simulink library "BibFHDO"  (R2025b)
settings: Solver=VariableStepAuto  StartTime=0.0  StopTime=10.0  RelTol=1e-3
libraries: $bdroot x16, BibSpielo x3, Bibliothek_FHDO_V1 x2
settings Model: Creator=henni  LastModifiedBy=henni

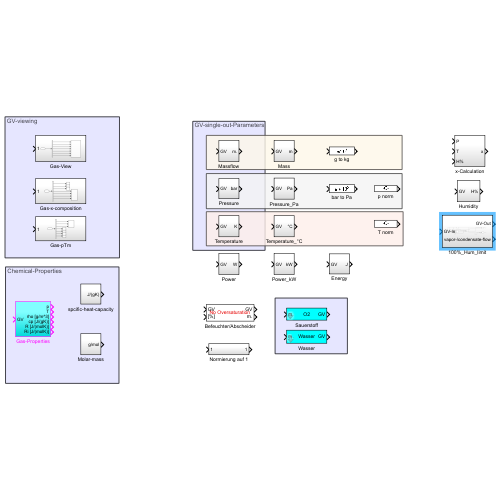
[thumbnail: Simulink's stored preview of the top-level diagram]
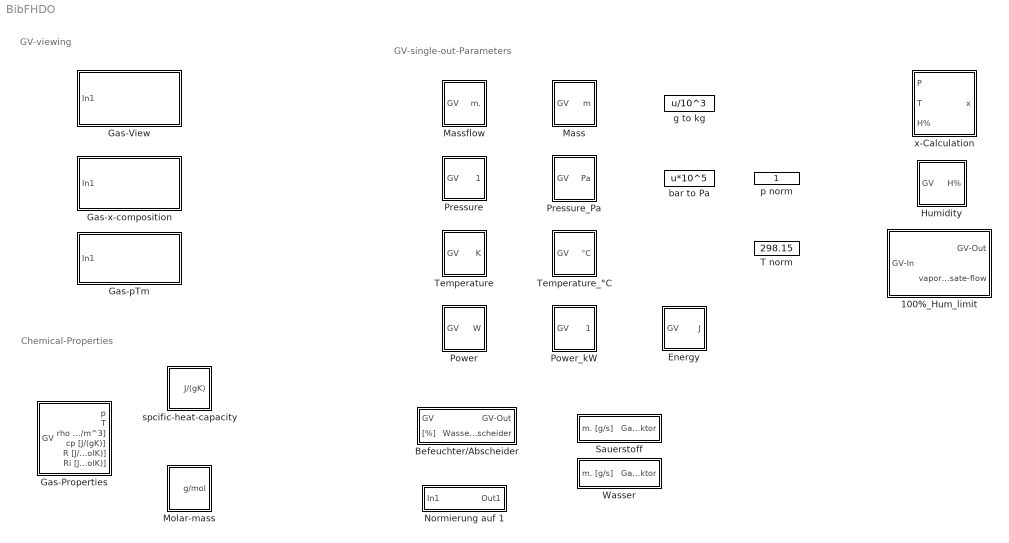
== system BibFHDO ==
  note: Chemical-Properties
  note: GV-viewing
  note: GV-single-out-Parameters
  100%_Hum_limit : Subsystem
  Befeuchter/Abscheider : Subsystem
      mask Display:
      | color('red')
      | disp('No Oversaturation');
      | 
      | color('black')
      | port_label('output', 1, 'GV')
      | port_label('output', 2, 'm.')
      | port_label('input', 1, 'GV')
      | port_label('input', 2, '[%]')
  Energy : Subsystem
  Gas-Properties : Subsystem
  Gas-View : Subsystem
  Gas-pTm : Subsystem
  Gas-x-composition : Subsystem
  Humidity : Subsystem
  Mass : Subsystem
  Massflow : Subsystem
  Molar-mass : Subsystem
  Normierung auf 1 : Subsystem
  Power : Subsystem
  Power_kW : Subsystem
  Pressure : Subsystem
  Pressure_Pa : Subsystem
  Sauerstoff : Subsystem  mask{p=1, T=25}
      mask prompts: p "p [bar]"; T "T [°C]"
      mask Display:
      | disp('O2')
      | 
      | port_label ('input', 1, 'm.')
      | port_label ('output', 1, 'GV')
  T norm : Constant  Value=298.15
  Temperature : Subsystem
  Temperature_°C : Subsystem
  Wasser : Subsystem  mask{p=1, T=25}
      mask prompts: p "p [bar]"; T "T [°C]"
      mask Display:
      | disp('Wasser')
      | 
      | port_label ('input', 1, 'm.')
      | port_label ('output', 1, 'GV')
  bar to Pa : Fcn  Expr=u*10^5
  g to kg : Fcn  Expr=u/10^3
  p norm : Constant
  spcific-heat-capacity : Subsystem
  x-Calculation : Subsystem

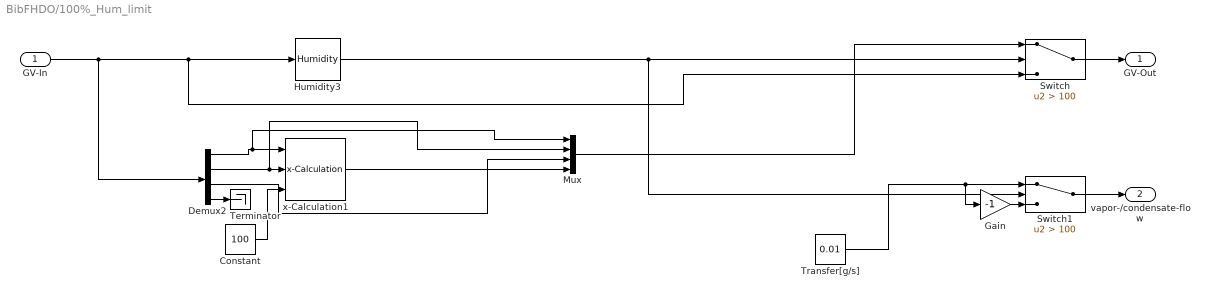
== system BibFHDO/100%_Hum_limit ==
  GV-In : Inport
  Constant : Constant  Value=100
  Demux2 : Demux  Outputs=[1 1 1 4]
  Gain : Gain  Gain=-1
  Humidity3 : $bdroot/Humidity  SystemSampleTime=-1  VariantActivationTime=update diagram  EmptyChoice=off  PassThrough=off  PassThroughVariantControl=(default)  EmptyChoiceVariantControl=(default)  AllowFlexibleInterface=on  Latency=0  AutoFrameSizeCalculation=off
  Mux : Mux  Inputs=[1 1 1 4]
  Switch : Switch  Criteria=u2 > Threshold  Threshold=100  SaturateOnIntegerOverflow=off  InputSameDT=off
  Switch1 : Switch  Criteria=u2 > Threshold  Threshold=100  SaturateOnIntegerOverflow=off  InputSameDT=off
  Terminator : Terminator
  Transfer[g/s] : Constant  Value=0.01
  x-Calculation1 : $bdroot/x-Calculation  SystemSampleTime=-1  VariantActivationTime=update diagram  EmptyChoice=off  PassThrough=off  PassThroughVariantControl=(default)  EmptyChoiceVariantControl=(default)  AllowFlexibleInterface=on  Latency=0  AutoFrameSizeCalculation=off
  GV-Out : Outport
  vapor-/condensate-flow : Outport  Port=2
  wires:
  Transfer[g/s]/1 -> Gain/1, Switch1/1
  Gain/1 -> Switch1/3
  Switch1/1 -> vapor-/condensate-flow/1
  x-Calculation1/1 -> Mux/4
  Switch/1 -> GV-Out/1
  Demux2/1 -> x-Calculation1/1, Mux/1
  Demux2/3 -> Mux/3
  Demux2/4 -> Terminator/1
  Demux2/2 -> x-Calculation1/2, Mux/2
  Humidity3/1 -> Switch/2, Switch1/2
  GV-In/1 -> Switch/3, Humidity3/1, Demux2/1
  Mux/1 -> Switch/1
  Constant/1 -> x-Calculation1/3

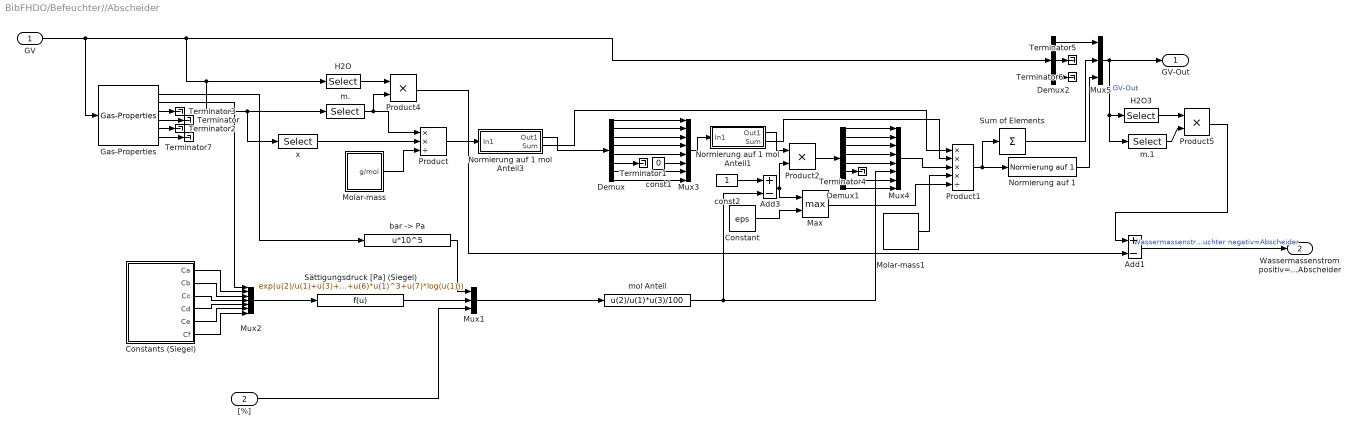
== system BibFHDO/Befeuchter//Abscheider ==
  GV : Inport
  "[%]" : Inport  Port=2
  Add1 : Sum  Inputs=+-
  Add3 : Sum  Inputs=+-
  Constant : Constant  Value=eps
  Constants (Siegel) : Subsystem
  Demux : Demux  Outputs=8
  Demux1 : Demux  Outputs=8
  Demux2 : Demux  Outputs=[2 1 8]
  Gas-Properties : $bdroot/Gas-Properties  SystemSampleTime=-1  VariantActivationTime=update diagram  EmptyChoice=off  PassThrough=off  PassThroughVariantControl=(default)  EmptyChoiceVariantControl=(default)  AllowFlexibleInterface=on  Latency=0  AutoFrameSizeCalculation=off
  H2O : Selector  InputPortWidth=11  IndexOptions=Index vector (dialog)  Indices=9  OutputSizes=1
  H2O3 : Selector  InputPortWidth=11  IndexOptions=Index vector (dialog)  Indices=9  OutputSizes=1
  Max : MinMax  Function=max  Inputs=2
  Molar-mass : Subsystem
  Molar-mass1 : $bdroot/Molar-mass  SystemSampleTime=-1  VariantActivationTime=update diagram  EmptyChoice=off  PassThrough=off  PassThroughVariantControl=(default)  EmptyChoiceVariantControl=(default)  AllowFlexibleInterface=on  Latency=0  AutoFrameSizeCalculation=off
  Mux1 : Mux  Inputs=3
  Mux2 : Mux  Inputs=7
  Mux3 : Mux  Inputs=8
  Mux4 : Mux  Inputs=8
  Mux5 : Mux  Inputs=3
  Normierung auf 1 : $bdroot/Normierung auf 1  SystemSampleTime=-1  VariantActivationTime=update diagram  EmptyChoice=off  PassThrough=off  PassThroughVariantControl=(default)  EmptyChoiceVariantControl=(default)  AllowFlexibleInterface=on  Latency=0  AutoFrameSizeCalculation=off
  Normierung auf 1 mol Anteil1 : Subsystem
  Normierung auf 1 mol Anteil3 : Subsystem
  Product : Product  Inputs=**/  RndMeth=Zero
  Product1 : Product  Inputs=****/  RndMeth=Zero
  Product2 : Product  RndMeth=Zero
  Product4 : Product  RndMeth=Zero
  Product5 : Product  RndMeth=Zero
  Sum of Elements : Sum  Inputs=+
  Sättigungsdruck [Pa] (Siegel) : Fcn  Expr=exp(u(2)/u(1)+u(3)+u(4)*u(1)+u(5)*u(1)^2+u(6)*u(1)^3+u(7)*log(u(1)))
  Terminator{,1..7} (8 alike) : Terminator
  "bar -> Pa" : Fcn  Expr=u*10^5
  const1 : Constant  Value=0
  const2 : Constant
  m. : Selector  InputPortWidth=11  IndexOptions=Index vector (dialog)  Indices=3  OutputSizes=1
  m.1 : Selector  InputPortWidth=11  IndexOptions=Index vector (dialog)  Indices=3  OutputSizes=1
  mol Anteil : Fcn  Expr=u(2)/u(1)*u(3)/100
  x : Selector  InputPortWidth=11  IndexOptions=Index vector (dialog)  Indices=[4 5 6 7 8 9 10 11]  OutputSizes=1
  GV-Out : Outport
  Wassermassenstrom positiv=Befeuchter negativ=Abscheider : Outport  Port=2
  wires:
  Product1/1 -> Normierung auf 1/1, Sum of Elements/1
  Sättigungsdruck [Pa] (Siegel)/1 -> Mux1/2
  Demux1/2 -> Mux4/2
  Gas-Properties/6 -> Terminator7/1
  Constants (Siegel)/5(Ce) -> Mux2/6
  Demux/2 -> Mux3/2
  Constants (Siegel)/1(Ca) -> Mux2/2
  Demux2/1 -> Mux5/1
  Demux/3 -> Mux3/3
  Molar-mass/1(g/mol) -> Product/3
  Mux3/1 -> Normierung auf 1 mol Anteil1/1(In1)
  GV/1 -> Gas-Properties/1, Demux2/1, m./1, x/1, H2O/1
  Product4/1 -> Add1/2
  Normierung auf 1 mol Anteil1/1(Out1) -> Product2/1
  Gas-Properties/1 -> "bar -> Pa"/1
  Constants (Siegel)/6(Cf) -> Mux2/7
  Normierung auf 1/1 -> Mux5/3
  const2/1 -> Add3/1
  Demux1/4 -> Mux4/4
  Gas-Properties/2 -> Mux2/1
  Demux1/1 -> Mux4/1
  Demux1/5 -> Mux4/5
  Constants (Siegel)/2(Cb) -> Mux2/3
  Demux/8 -> Mux3/8
  Demux/6 -> Terminator1/1
  Product2/1 -> Demux1/1
  Demux/1 -> Mux3/1
  Molar-mass1/1 -> Product1/4
  Mux2/1 -> Sättigungsdruck [Pa] (Siegel)/1
  Demux1/7 -> Mux4/7
  Add3/1 -> Max/1, Product2/2
  Mux5/1 -> m.1/1, H2O3/1, GV-Out/1  "GV-Out"
  Add1/1 -> Wassermassenstrom positiv=Befeuchter negativ=Abscheider/1  "Wassermassenstrom positiv=Befeuchter negativ=Abscheider"
  Demux1/3 -> Mux4/3
  Sum of Elements/1 -> Mux5/2
  m.1/1 -> Product5/2
  Product5/1 -> Add1/1
  Product/1 -> Normierung auf 1 mol Anteil3/1(In1)
  Demux2/2 -> Terminator5/1
  Gas-Properties/3 -> Terminator3/1
  x/1 -> Product/2
  const1/1 -> Mux3/6
  H2O/1 -> Product4/1
  mol Anteil/1 -> Mux4/6, Add3/2
  Demux/7 -> Mux3/7
  H2O3/1 -> Product5/1
  Constants (Siegel)/3(Cc) -> Mux2/4
  Mux1/1 -> mol Anteil/1
  Normierung auf 1 mol Anteil1/2(Sum) -> Product1/2
  "bar -> Pa"/1 -> Mux1/1
  Demux1/6 -> Terminator4/1
  m./1 -> Product/1, Product4/2
  Mux4/1 -> Product1/3
  Demux2/3 -> Terminator6/1
  Demux1/8 -> Mux4/8
  Demux/4 -> Mux3/4
  Demux/5 -> Mux3/5
  Normierung auf 1 mol Anteil3/1(Out1) -> Demux/1
  Normierung auf 1 mol Anteil3/2(Sum) -> Product1/1
  Constants (Siegel)/4(Cd) -> Mux2/5
  Gas-Properties/4 -> Terminator/1
  Gas-Properties/5 -> Terminator2/1
  "[%]"/1 -> Mux1/3
  Constant/1 -> Max/2
  Max/1 -> Product1/5

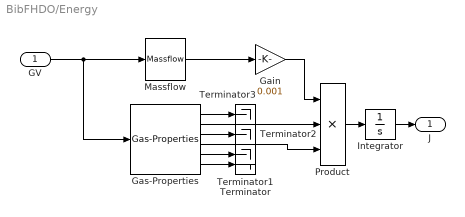
== system BibFHDO/Energy ==
  GV : Inport
  Gain : Gain  Gain=0.001
  Gas-Properties : $bdroot/Gas-Properties  SystemSampleTime=-1  VariantActivationTime=update diagram  EmptyChoice=off  PassThrough=off  PassThroughVariantControl=(default)  EmptyChoiceVariantControl=(default)  AllowFlexibleInterface=on  Latency=0  AutoFrameSizeCalculation=off
  Integrator : Integrator
  Massflow : $bdroot/Massflow  SystemSampleTime=-1  VariantActivationTime=update diagram  EmptyChoice=off  PassThrough=off  PassThroughVariantControl=(default)  EmptyChoiceVariantControl=(default)  AllowFlexibleInterface=on  Latency=0  AutoFrameSizeCalculation=off
  Product : Product  Inputs=3
  Terminator{,1..3} (4 alike) : Terminator
  J : Outport
  wires:
  GV/1 -> Gas-Properties/1, Massflow/1
  Gas-Properties/5 -> Terminator1/1
  Gas-Properties/2 -> Product/2
  Gas-Properties/3 -> Terminator2/1
  Gas-Properties/1 -> Terminator3/1
  Gas-Properties/4 -> Product/3
  Massflow/1 -> Gain/1
  Gas-Properties/6 -> Terminator/1
  Gain/1 -> Product/1
  Product/1 -> Integrator/1
  Integrator/1 -> J/1

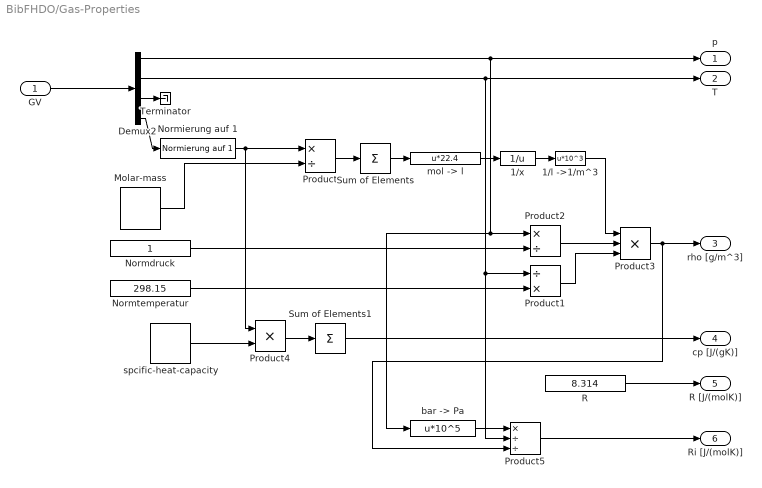
== system BibFHDO/Gas-Properties ==
  GV : Inport
  1/l ->1/m^3 : Fcn  Expr=u*10^3
  1/x : Fcn  Expr=1/u
  Demux2 : Demux  Outputs=[1 1 1 4]
  Molar-mass : BibSpielo/Molar-mass  SystemSampleTime=-1  VariantActivationTime=update diagram  EmptyChoice=off  PassThrough=off  PassThroughVariantControl=(default)  EmptyChoiceVariantControl=(default)  AllowFlexibleInterface=on  Latency=0  AutoFrameSizeCalculation=off
  Normdruck : Constant
  Normierung auf 1 : BibSpielo/Normierung auf 1  SystemSampleTime=-1  VariantActivationTime=update diagram  EmptyChoice=off  PassThrough=off  PassThroughVariantControl=(default)  EmptyChoiceVariantControl=(default)  AllowFlexibleInterface=on  Latency=0  AutoFrameSizeCalculation=off
  Normtemperatur : Constant  Value=298.15
  Product : Product  Inputs=*/  RndMeth=Zero
  Product1 : Product  Inputs=/*  RndMeth=Zero
  Product2 : Product  Inputs=*/  RndMeth=Zero
  Product3 : Product  Inputs=3  RndMeth=Zero
  Product4 : Product  RndMeth=Zero
  Product5 : Product  Inputs=*//
  R : Constant  Value=8.314
  Sum of Elements : Sum  Inputs=+
  Sum of Elements1 : Sum  Inputs=+
  Terminator : Terminator
  "bar -> Pa" : Fcn  Expr=u*10^5
  "mol -> l" : Fcn  Expr=u*22.4
  spcific-heat-capacity : BibSpielo/spcific-heat-capacity  SystemSampleTime=-1  VariantActivationTime=update diagram  EmptyChoice=off  PassThrough=off  PassThroughVariantControl=(default)  EmptyChoiceVariantControl=(default)  AllowFlexibleInterface=on  Latency=0  AutoFrameSizeCalculation=off
  p : Outport
  T : Outport  Port=2
  rho [g/m^3] : Outport  Port=3
  cp [J/(gK)] : Outport  Port=4
  R [J/(molK)] : Outport  Port=5
  Ri [J/(molK)] : Outport  Port=6
  wires:
  1/l ->1/m^3/1 -> Product3/1
  Product2/1 -> Product3/2
  1/x/1 -> 1/l ->1/m^3/1
  R/1 -> R [J/(molK)]/1
  Demux2/1 -> p/1, Product2/1, "bar -> Pa"/1
  GV/1 -> Demux2/1
  spcific-heat-capacity/1 -> Product4/2
  "mol -> l"/1 -> 1/x/1
  Product1/1 -> Product3/3
  Molar-mass/1 -> Product/2
  Normtemperatur/1 -> Product1/2
  Normierung auf 1/1 -> Product/1, Product4/1
  Sum of Elements/1 -> "mol -> l"/1
  Demux2/3 -> Terminator/1
  "bar -> Pa"/1 -> Product5/1
  Product4/1 -> Sum of Elements1/1
  Demux2/2 -> T/1, Product5/2, Product1/1
  Sum of Elements1/1 -> cp [J/(gK)]/1
  Product/1 -> Sum of Elements/1
  Product3/1 -> rho [g/m^3]/1, Product5/3
  Normdruck/1 -> Product2/2
  Demux2/4 -> Normierung auf 1/1
  Product5/1 -> Ri [J/(molK)]/1

== system BibFHDO/Gas-View ==
  In1 : Inport
  Demux : Demux  Outputs=7
  Scope : Scope  NumInputPorts=7
  wires:
  In1/1 -> Demux/1
  Demux/5 -> Scope/5  "H2O"
  Demux/6 -> Scope/6  "O2"
  Demux/4 -> Scope/4  "H2%"
  Demux/7 -> Scope/7  "N2"
  Demux/1 -> Scope/1  "Druck"
  Demux/2 -> Scope/2  "Temperatur"
  Demux/3 -> Scope/3  "Massenstrom"

== system BibFHDO/Gas-pTm ==
  In1 : Inport
  Demux : Demux  Outputs=7
  Scope : Scope  NumInputPorts=3
      settings: DataLoggingVariableName=ScopeData2
  Terminator{,1..3} (4 alike) : Terminator
  wires:
  Demux/6 -> Terminator1/1
  In1/1 -> Demux/1
  Demux/3 -> Scope/3  "m"
  Demux/1 -> Scope/1  "p"
  Demux/2 -> Scope/2  "T"
  Demux/4 -> Terminator3/1
  Demux/5 -> Terminator2/1
  Demux/7 -> Terminator/1

== system BibFHDO/Gas-x-composition ==
  In1 : Inport
  Demux : Demux  Outputs=7
  Scope : Scope  NumInputPorts=4
  Terminator : Terminator
  Terminator1 : Terminator
  Terminator2 : Terminator
  wires:
  Demux/6 -> Scope/3  "O2"
  Demux/7 -> Scope/4  "N2"
  In1/1 -> Demux/1
  Demux/2 -> Terminator1/1
  Demux/1 -> Terminator/1
  Demux/4 -> Scope/1  "H2"
  Demux/3 -> Terminator2/1
  Demux/5 -> Scope/2  "H2O"

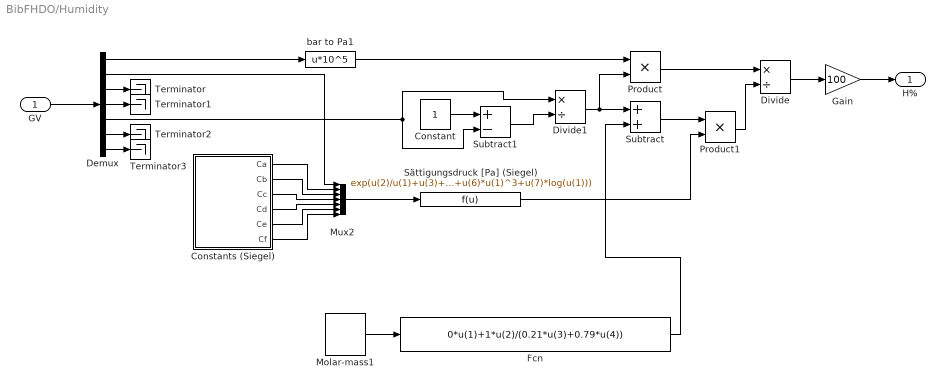
== system BibFHDO/Humidity ==
  GV : Inport
  Constant : Constant
  Constants (Siegel) : Subsystem
  Demux : Demux  Outputs=7
  Divide : Product  Inputs=*/
  Divide1 : Product  Inputs=*/
  Fcn : Fcn  Expr=0*u(1)+1*u(2)/(0.21*u(3)+0.79*u(4))
  Gain : Gain  Gain=100
  Molar-mass1 : $bdroot/Molar-mass  SystemSampleTime=-1  VariantActivationTime=update diagram  EmptyChoice=off  PassThrough=off  PassThroughVariantControl=(default)  EmptyChoiceVariantControl=(default)  AllowFlexibleInterface=on  Latency=0  AutoFrameSizeCalculation=off
  Mux2 : Mux  Inputs=7
  Product : Product
  Product1 : Product
  Subtract : Sum
  Subtract1 : Sum  Inputs=+-
  Sättigungsdruck [Pa] (Siegel) : Fcn  Expr=exp(u(2)/u(1)+u(3)+u(4)*u(1)+u(5)*u(1)^2+u(6)*u(1)^3+u(7)*log(u(1)))
  Terminator{,1..3} (4 alike) : Terminator
  bar to Pa1 : Fcn  Expr=u*10^5
  H% : Outport
  wires:
  Demux/2 -> Mux2/1
  Constants (Siegel)/2(Cb) -> Mux2/3
  Mux2/1 -> Sättigungsdruck [Pa] (Siegel)/1
  Fcn/1 -> Subtract/2
  Demux/5 -> Divide1/1, Subtract1/2
  GV/1 -> Demux/1
  Demux/6 -> Terminator2/1
  Demux/3 -> Terminator/1
  Molar-mass1/1 -> Fcn/1
  bar to Pa1/1 -> Product/1
  Divide/1 -> Gain/1
  Demux/1 -> bar to Pa1/1
  Demux/4 -> Terminator1/1
  Demux/7 -> Terminator3/1
  Constants (Siegel)/4(Cd) -> Mux2/5
  Constants (Siegel)/6(Cf) -> Mux2/7
  Constants (Siegel)/3(Cc) -> Mux2/4
  Constants (Siegel)/5(Ce) -> Mux2/6
  Constants (Siegel)/1(Ca) -> Mux2/2
  Product/1 -> Divide/1
  Subtract/1 -> Product1/1
  Sättigungsdruck [Pa] (Siegel)/1 -> Product1/2
  Product1/1 -> Divide/2
  Gain/1 -> H%/1
  Constant/1 -> Subtract1/1
  Subtract1/1 -> Divide1/2
  Divide1/1 -> Product/2, Subtract/1

== system BibFHDO/Mass ==
  GV : Inport
  Integrator : Integrator
  Massflow : $bdroot/Massflow  SystemSampleTime=-1  VariantActivationTime=update diagram  EmptyChoice=off  PassThrough=off  PassThroughVariantControl=(default)  EmptyChoiceVariantControl=(default)  AllowFlexibleInterface=on  Latency=0  AutoFrameSizeCalculation=off
  m : Outport
  wires:
  Massflow/1 -> Integrator/1
  GV/1 -> Massflow/1
  Integrator/1 -> m/1

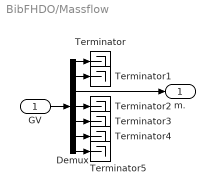
== system BibFHDO/Massflow ==
  GV : Inport
  Demux : Demux  Outputs=7
  Terminator{,1..5} (6 alike) : Terminator
  m. : Outport
  wires:
  Demux/2 -> Terminator1/1
  GV/1 -> Demux/1
  Demux/4 -> Terminator2/1
  Demux/6 -> Terminator4/1
  Demux/5 -> Terminator3/1
  Demux/1 -> Terminator/1
  Demux/7 -> Terminator5/1
  Demux/3 -> m./1

== system BibFHDO/Molar-mass ==
  note: VDI Wärmeatlas
      | Normbedingungen
      | p=1bar
      | T=298.15K
  H2 : Constant  Value=2.016
  H2O : Constant  Value=18.015
  Mux : Mux
  N2 : Constant  Value=28.013
  O2 : Constant  Value=31.999
  g/mol : Outport
  wires:
  H2O/1 -> Mux/2
  N2/1 -> Mux/4
  O2/1 -> Mux/3
  Mux/1 -> g/mol/1
  H2/1 -> Mux/1

== system BibFHDO/Normierung auf 1 ==
  In1 : Inport
  Product : Product  Inputs=*/  RndMeth=Zero
  Sum of Elements : Sum  Inputs=+
  Out1 : Outport
  wires:
  Sum of Elements/1 -> Product/2
  In1/1 -> Product/1, Sum of Elements/1
  Product/1 -> Out1/1

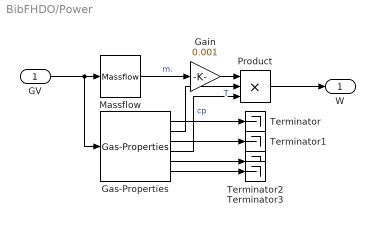
== system BibFHDO/Power ==
  GV : Inport
  Gain : Gain  Gain=0.001
  Gas-Properties : $bdroot/Gas-Properties  SystemSampleTime=-1  VariantActivationTime=update diagram  EmptyChoice=off  PassThrough=off  PassThroughVariantControl=(default)  EmptyChoiceVariantControl=(default)  AllowFlexibleInterface=on  Latency=0  AutoFrameSizeCalculation=off
  Massflow : $bdroot/Massflow  SystemSampleTime=-1  VariantActivationTime=update diagram  EmptyChoice=off  PassThrough=off  PassThroughVariantControl=(default)  EmptyChoiceVariantControl=(default)  AllowFlexibleInterface=on  Latency=0  AutoFrameSizeCalculation=off
  Product : Product  Inputs=3
  Terminator{,1..3} (4 alike) : Terminator
  W : Outport
  wires:
  Massflow/1 -> Gain/1  "m."
  Gas-Properties/3 -> Terminator1/1
  GV/1 -> Gas-Properties/1, Massflow/1
  Gas-Properties/2 -> Product/2  "T"
  Gas-Properties/1 -> Terminator/1
  Gas-Properties/4 -> Product/3  "cp"
  Gas-Properties/5 -> Terminator2/1
  Gas-Properties/6 -> Terminator3/1
  Product/1 -> W/1
  Gain/1 -> Product/1

== system BibFHDO/Power_kW ==
  GV : Inport
  Gain : Gain  Gain=1000
  Power : $bdroot/Power  SystemSampleTime=-1  VariantActivationTime=update diagram  EmptyChoice=off  PassThrough=off  PassThroughVariantControl=(default)  EmptyChoiceVariantControl=(default)  AllowFlexibleInterface=on  Latency=0  AutoFrameSizeCalculation=off
  kW : Outport
  wires:
  GV/1 -> Power/1
  Gain/1 -> kW/1
  Power/1 -> Gain/1

== system BibFHDO/Pressure ==
  GV : Inport
  Demux : Demux  Outputs=7
  Terminator{1..6} (6 alike) : Terminator
  bar : Outport
  wires:
  Demux/3 -> Terminator6/1
  Demux/7 -> Terminator5/1
  Demux/6 -> Terminator4/1
  GV/1 -> Demux/1
  Demux/4 -> Terminator2/1
  Demux/2 -> Terminator1/1
  Demux/5 -> Terminator3/1
  Demux/1 -> bar/1

== system BibFHDO/Pressure_Pa ==
  GV : Inport
  Multiply : Gain  Gain=100000
  Pressure : $bdroot/Pressure  SystemSampleTime=-1  VariantActivationTime=update diagram  EmptyChoice=off  PassThrough=off  PassThroughVariantControl=(default)  EmptyChoiceVariantControl=(default)  AllowFlexibleInterface=on  Latency=0  AutoFrameSizeCalculation=off
  Pa : Outport
  wires:
  Pressure/1 -> Multiply/1
  GV/1 -> Pressure/1
  Multiply/1 -> Pa/1

== system BibFHDO/Sauerstoff ==
  m. [g/s] : Inport
  Mux : Mux
  Normierung auf 2 : Bibliothek_FHDO_V1/Sauerstoff/Normierung auf 1  SystemSampleTime=-1  VariantActivationTime=update diagram  EmptyChoice=off  PassThrough=off  PassThroughVariantControl=(default)  EmptyChoiceVariantControl=(default)  AllowFlexibleInterface=on  Latency=0  AutoFrameSizeCalculation=off
  Saturation : Saturate  UpperLimit=inf  LowerLimit=eps
  T : Constant  Value=273.15+T
  p : Constant  Value=p
  x : Constant  Value=[0 0 1 0]
  Gasvektor : Outport
  wires:
  p/1 -> Mux/1
  x/1 -> Normierung auf 2/1
  Normierung auf 2/1 -> Mux/4
  Mux/1 -> Gasvektor/1  "Gasvektor"
  T/1 -> Mux/2
  m. [g/s]/1 -> Saturation/1
  Saturation/1 -> Mux/3

== system BibFHDO/Temperature ==
  GV : Inport
  Demux : Demux  Outputs=7
  Terminator{,1..5} (6 alike) : Terminator
  K : Outport
  wires:
  Demux/3 -> Terminator1/1
  Demux/7 -> Terminator5/1
  GV/1 -> Demux/1
  Demux/4 -> Terminator2/1
  Demux/1 -> Terminator/1
  Demux/6 -> Terminator4/1
  Demux/5 -> Terminator3/1
  Demux/2 -> K/1

== system BibFHDO/Temperature_°C ==
  GV : Inport
  Add Constant : Bias  Bias=273.15  SaturateOnIntegerOverflow=off
  Temperature : $bdroot/Temperature  SystemSampleTime=-1  VariantActivationTime=update diagram  EmptyChoice=off  PassThrough=off  PassThroughVariantControl=(default)  EmptyChoiceVariantControl=(default)  AllowFlexibleInterface=on  Latency=0  AutoFrameSizeCalculation=off
  °C : Outport
  wires:
  GV/1 -> Temperature/1
  Temperature/1 -> Add Constant/1
  Add Constant/1 -> °C/1

== system BibFHDO/Wasser ==
  m. [g/s] : Inport
  Mux : Mux
  Normierung auf 2 : Bibliothek_FHDO_V1/Wasser/Normierung auf 1  SystemSampleTime=-1  VariantActivationTime=update diagram  EmptyChoice=off  PassThrough=off  PassThroughVariantControl=(default)  EmptyChoiceVariantControl=(default)  AllowFlexibleInterface=on  Latency=0  AutoFrameSizeCalculation=off
  Saturation : Saturate  UpperLimit=inf  LowerLimit=eps
  T : Constant  Value=273.15+T
  p : Constant  Value=p
  x : Constant  Value=[0 1 0 0]
  Gasvektor : Outport
  wires:
  p/1 -> Mux/1
  T/1 -> Mux/2
  Normierung auf 2/1 -> Mux/4
  Saturation/1 -> Mux/3
  x/1 -> Normierung auf 2/1
  Mux/1 -> Gasvektor/1  "Gasvektor"
  m. [g/s]/1 -> Saturation/1

== system BibFHDO/spcific-heat-capacity ==
  note: VDI Wärmeatlas
      | Normbedingungen
      | p=1bar
      | T=298.15K
  H2 : Constant  Value=14.286
  H2O : Constant  Value=1.879
  Mux : Mux
  N2 : Constant  Value=1.037
  O2 : Constant  Value=0.927
  J/(gK) : Outport
  wires:
  N2/1 -> Mux/4
  H2O/1 -> Mux/2
  O2/1 -> Mux/3
  Mux/1 -> J/(gK)/1
  H2/1 -> Mux/1

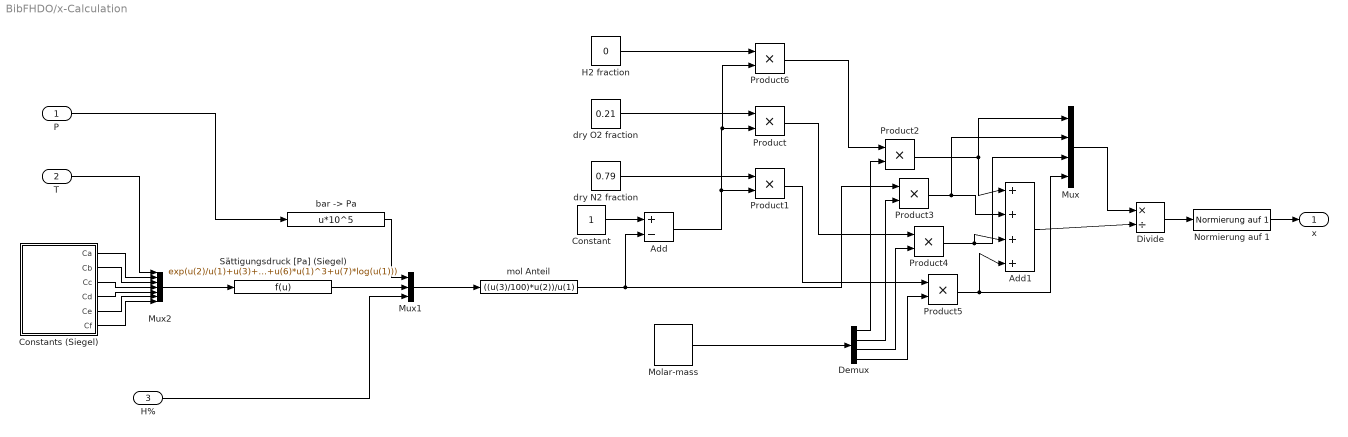
== system BibFHDO/x-Calculation ==
  P : Inport
  T : Inport  Port=2
  H% : Inport  Port=3
  Add : Sum  Inputs=+-
  Add1 : Sum  Inputs=++++
  Constant : Constant
  Constants (Siegel) : Subsystem
  Demux : Demux
  Divide : Product  Inputs=*/
  H2 fraction : Constant  Value=0
  Molar-mass : $bdroot/Molar-mass  SystemSampleTime=-1  VariantActivationTime=update diagram  EmptyChoice=off  PassThrough=off  PassThroughVariantControl=(default)  EmptyChoiceVariantControl=(default)  AllowFlexibleInterface=on  Latency=0  AutoFrameSizeCalculation=off
  Mux : Mux
  Mux1 : Mux  Inputs=3
  Mux2 : Mux  Inputs=7
  Normierung auf 1 : $bdroot/Normierung auf 1  SystemSampleTime=-1  VariantActivationTime=update diagram  EmptyChoice=off  PassThrough=off  PassThroughVariantControl=(default)  EmptyChoiceVariantControl=(default)  AllowFlexibleInterface=on  Latency=0  AutoFrameSizeCalculation=off
  Product{,1..6} (7 alike) : Product
  Sättigungsdruck [Pa] (Siegel) : Fcn  Expr=exp(u(2)/u(1)+u(3)+u(4)*u(1)+u(5)*u(1)^2+u(6)*u(1)^3+u(7)*log(u(1)))
  "bar -> Pa" : Fcn  Expr=u*10^5
  dry N2 fraction : Constant  Value=0.79
  dry O2 fraction : Constant  Value=0.21
  mol Anteil : Fcn  Expr=((u(3)/100)*u(2))/u(1)
  x : Outport
  wires:
  Constants (Siegel)/4(Cd) -> Mux2/5
  Constants (Siegel)/3(Cc) -> Mux2/4
  Constants (Siegel)/6(Cf) -> Mux2/7
  Constants (Siegel)/5(Ce) -> Mux2/6
  Constants (Siegel)/1(Ca) -> Mux2/2
  "bar -> Pa"/1 -> Mux1/1
  Sättigungsdruck [Pa] (Siegel)/1 -> Mux1/2
  Mux2/1 -> Sättigungsdruck [Pa] (Siegel)/1
  Constants (Siegel)/2(Cb) -> Mux2/3
  Mux1/1 -> mol Anteil/1
  H%/1 -> Mux1/3
  mol Anteil/1 -> Product3/1, Add/2
  P/1 -> "bar -> Pa"/1
  dry O2 fraction/1 -> Product/1
  dry N2 fraction/1 -> Product1/1
  Constant/1 -> Add/1
  H2 fraction/1 -> Product6/1
  Product1/1 -> Product5/1
  Product/1 -> Product4/1
  Molar-mass/1 -> Demux/1
  Demux/1 -> Product2/2
  Demux/2 -> Product3/2
  Demux/4 -> Product5/2
  Demux/3 -> Product4/2
  Product2/1 -> Mux/1, Add1/1
  Product3/1 -> Mux/2, Add1/2
  Product4/1 -> Mux/3, Add1/3
  Product5/1 -> Mux/4, Add1/4
  Mux/1 -> Divide/1
  Divide/1 -> Normierung auf 1/1
  Add1/1 -> Divide/2
  T/1 -> Mux2/1
  Normierung auf 1/1 -> x/1
  Product6/1 -> Product2/1
  Add/1 -> Product6/2, Product/2, Product1/2

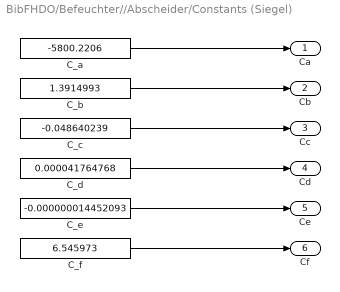
== system BibFHDO/Befeuchter//Abscheider/Constants (Siegel) ==
  C_a : Constant  Value=-5800.2206
  C_b : Constant  Value=1.3914993
  C_c : Constant  Value=-0.048640239
  C_d : Constant  Value=0.000041764768
  C_e : Constant  Value=-0.000000014452093
  C_f : Constant  Value=6.545973
  Ca : Outport
  Cb : Outport  Port=2
  Cc : Outport  Port=3
  Cd : Outport  Port=4
  Ce : Outport  Port=5
  Cf : Outport  Port=6
  wires:
  C_f/1 -> Cf/1
  C_a/1 -> Ca/1
  C_e/1 -> Ce/1
  C_d/1 -> Cd/1
  C_c/1 -> Cc/1
  C_b/1 -> Cb/1

== system BibFHDO/Befeuchter//Abscheider/Molar-mass ==
  note: VDI Wärmeatlas
      | Normbedingungen
      | p=1bar
      | T=298.15K
  H2 : Constant  Value=2.016
  H2O : Constant  Value=18.015
  Mux : Mux
  N2 : Constant  Value=28.013
  O2 : Constant  Value=31.999
  g/mol : Outport
  wires:
  H2O/1 -> Mux/2
  N2/1 -> Mux/4
  O2/1 -> Mux/3
  Mux/1 -> g/mol/1
  H2/1 -> Mux/1

== system BibFHDO/Befeuchter//Abscheider/Normierung auf 1 mol Anteil1 ==
  In1 : Inport
  Mux : Mux  Inputs=8
  Product3 : Product  Inputs=*/  RndMeth=Zero
  Sum of Elements1 : Sum  Inputs=+
  Switch : Switch  Criteria=u2 > Threshold  SaturateOnIntegerOverflow=off  InputSameDT=off
  Out1 : Outport
  Sum : Outport  Port=2
  wires:
  Sum of Elements1/1 -> Mux/8, Mux/7, Mux/6, Mux/5, Mux/4, Mux/3, Mux/2, Mux/1, Sum/1, Switch/2, Product3/2
  In1/1 -> Sum of Elements1/1, Product3/1
  Mux/1 -> Switch/3
  Product3/1 -> Switch/1
  Switch/1 -> Out1/1

== system BibFHDO/Befeuchter//Abscheider/Normierung auf 1 mol Anteil3 ==
  In1 : Inport
  Mux : Mux  Inputs=8
  Product3 : Product  Inputs=*/  RndMeth=Zero
  Sum of Elements1 : Sum  Inputs=+
  Switch : Switch  Criteria=u2 > Threshold  SaturateOnIntegerOverflow=off  InputSameDT=off
  Out1 : Outport
  Sum : Outport  Port=2
  wires:
  In1/1 -> Product3/1, Sum of Elements1/1
  Switch/1 -> Out1/1
  Sum of Elements1/1 -> Mux/7, Mux/8, Mux/6, Mux/5, Mux/4, Mux/3, Mux/2, Mux/1, Sum/1, Switch/2, Product3/2
  Mux/1 -> Switch/3
  Product3/1 -> Switch/1

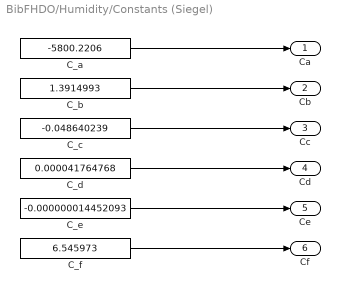
== system BibFHDO/Humidity/Constants (Siegel) ==
  C_a : Constant  Value=-5800.2206
  C_b : Constant  Value=1.3914993
  C_c : Constant  Value=-0.048640239
  C_d : Constant  Value=0.000041764768
  C_e : Constant  Value=-0.000000014452093
  C_f : Constant  Value=6.545973
  Ca : Outport
  Cb : Outport  Port=2
  Cc : Outport  Port=3
  Cd : Outport  Port=4
  Ce : Outport  Port=5
  Cf : Outport  Port=6
  wires:
  C_f/1 -> Cf/1
  C_a/1 -> Ca/1
  C_e/1 -> Ce/1
  C_d/1 -> Cd/1
  C_c/1 -> Cc/1
  C_b/1 -> Cb/1

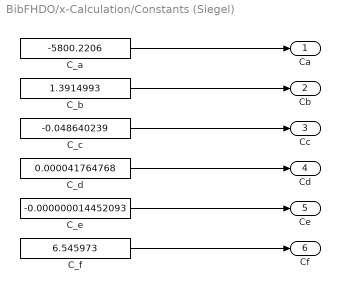
== system BibFHDO/x-Calculation/Constants (Siegel) ==
  C_a : Constant  Value=-5800.2206
  C_b : Constant  Value=1.3914993
  C_c : Constant  Value=-0.048640239
  C_d : Constant  Value=0.000041764768
  C_e : Constant  Value=-0.000000014452093
  C_f : Constant  Value=6.545973
  Ca : Outport
  Cb : Outport  Port=2
  Cc : Outport  Port=3
  Cd : Outport  Port=4
  Ce : Outport  Port=5
  Cf : Outport  Port=6
  wires:
  C_b/1 -> Cb/1
  C_c/1 -> Cc/1
  C_d/1 -> Cd/1
  C_e/1 -> Ce/1
  C_a/1 -> Ca/1
  C_f/1 -> Cf/1
